simulink library "lib_electric_machine2"  (Simulink 10.1)
settings: Solver=VariableStepAuto  StartTime=0.0  StopTime=10.0  RelTol=1e-3
undefined symbols (not defined in the file or in its folder): amb_tmp, fd_ratio, gb_ratio, gc_inertia, gc_map_spd, gc_map_trq, gc_max_crrnt, gc_max_trq, gc_outpwr_map, gc_overtrq_factor, gc_spd_scale, gc_trq_scale, mc_cp, mc_inertia, mc_init_tmp, mc_inpwr_map, mc_map_spd, mc_map_trq, mc_mass, mc_max_crrnt, mc_max_gen_trq, mc_max_trq, mc_overtrq_factor, mc_sarea, mc_spd_scale, mc_th_calc, mc_trq_scale, mc_tstat, veh_mass, wh_radius
undefined symbols (not defined in the file): logFlag
libraries: lib_electric_machine x1
(part 3 of 3)

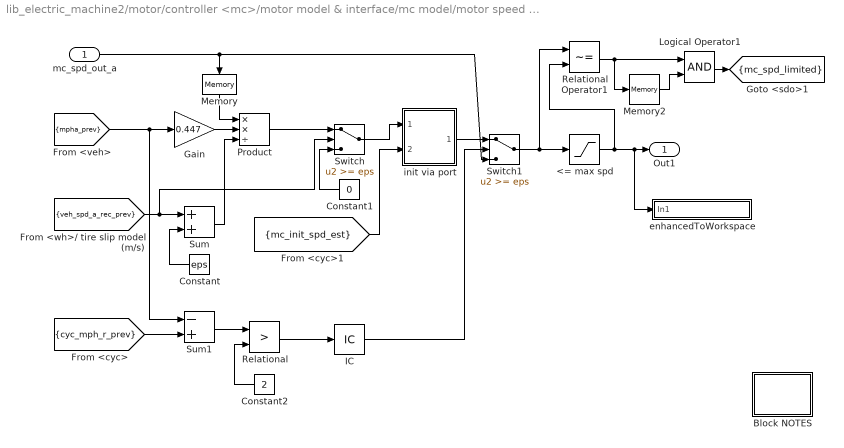
== system lib_electric_machine2/motor/controller <mc>/motor model & interface/mc model/motor speed estimator ==
  mc_spd_out_a : Inport
  <= max spd : Saturate  UpperLimit=max(mc_map_spd)*mc_spd_scale  LowerLimit=-inf
  Block NOTES : Subsystem
      mask Display: disp('Block\nNOTES')
  Constant : Constant  Value=eps
  Constant1 : Constant  Value=0
  Constant2 : Constant  Value=2
  Gain : Gain  Gain=0.447  SaturateOnIntegerOverflow=on
  IC : InitialCondition
  Logical Operator1 : Logic
  Memory : Memory
  Memory2 : Memory
  Product : Product  Inputs=**/  SaturateOnIntegerOverflow=on
  Relational : RelationalOperator  Operator=>  RndMeth=Nearest  InputSameDT=on
  Relational Operator1 : RelationalOperator  Operator=~=  RndMeth=Nearest  InputSameDT=on
  Sum : Sum  SaturateOnIntegerOverflow=on
  Sum1 : Sum  Inputs=-+  SaturateOnIntegerOverflow=on
  Switch : Switch  Threshold=eps  SaturateOnIntegerOverflow=on  InputSameDT=on
  Switch1 : Switch  Threshold=eps  SaturateOnIntegerOverflow=on  InputSameDT=on
  enhancedToWorkspace : Subsystem  mask(enhancedToWorkspace){generalName=generalName, specificName=spd_est, logFlag=logFlag}
      mask prompts: generalName "General Name [char-evaluated]"; specificName "Specific Name [char-literal]"; logFlag "Enable flag (1=on,0=off)"
      mask help: A wrapper for the Simulink "To Workspace" block that allows you to evaluate the name of the variable to log to workspace. This is useful to avoid the double logging errors that occur when you pull in two library models that attempt to log to the same variable.
      mask init:
      | enhancedToWsMaker
      settings: CopyFcn=breakLinkCopyFcn  ParentCloseFcn=breakLinkParCloseFcn
      mask Help:
      | <h2>Enhanced To Workspace Block</h2>
      | <h3>Parameters</h3>
      | <UL>
      | <li><b>General Name:</b> This is the more general name of the variable. Variables are saved to the workspace as <i>generalName_specificName</i>. Note that this is an evaluated variable. If you would like to type in the value directly, it must be surrounded with single quotes. Otherwise you can input the name of a variable containing a char string.</li>
      | <li><b>Specific Name:</b> This is the specific name of the variable. Note that this is input as a char literal (i.e., you don't need quotes).</li>
      | <li><b>Enable Flag:</b> This flag should have the value of 0 or 1. If 0, the variable will not be logged to the workspace. If 1, the variable will be logged. This is done so that variable logging can be turned off to improve speed.</li>
      | </ul>
      | <h3>Overview</h3>
      | <p>The enhanced to workspace block was put together to allow one to dynamically resolve variable names at run time in simulink. This is most powerful when used in conjunction with a masked subsystem to allow multiple instances of that masked subsytem to be used in the same model. The strategy is to set the generalName in the block mask which will allow the block to change the general name for all variable logging on the fly.
      | <h3>Helper Files</h3>
      | <p>Three m-files are required by the enhancedToWorkspace block. These files are located in the &lt; ADVISOR root &gt;/GUI directory :
      | <ul>
      | <li><i>enhancedToWsMaker.m</i> This file runs the mask initialization for the block</li>
      | <li><i>breakLinkCopyFcn.m</i> This file is used by the block callback when the simulink block is copied. It is necessary to break the link to the enhancedToWorkspace similar to the To Workspace block in order for it to be able to configure itself. (Try copying simulink's To Workspace block--it is impossible to make a link)</li>
      | <li><i>breakLinkParCloseFcn.m</i> This file is similar to the breakLinkCopyFcn and is used when a parent system is closed</li>
      | </ul>
      | <hr>
      | 
      | <p>Created 2003-Jan-21, Michael Patrick O'Keefe, NREL</p>
      mask Display: disp([generalName,'_',specificName])
  init via port : Subsystem
  Out1 : Outport
  tag scope: mc_spd_limited=scoped
  wires:
  Memory/1 -> Product/1
  [mc_init_spd_est] -> init via port/2(signal init)
  <= max spd/1 -> Relational Operator1/2, Out1/1, enhancedToWorkspace/1(In1)
  Switch1/1 -> Relational Operator1/1, <= max spd/1
  Relational Operator1/1 -> Memory2/1, Logical Operator1/1
  Logical Operator1/1 -> [mc_spd_limited]
  Memory2/1 -> Logical Operator1/2
  mc_spd_out_a/1 -> Memory/1, Switch1/3
  Product/1 -> Switch/1
  Sum/1 -> Product/3
  Gain/1 -> Product/2
  [veh_spd_a_rec_prev] -> Sum/1, Switch/2
  Constant1/1 -> Switch/3
  init via port/1(signal out) -> Switch1/1
  Constant/1 -> Sum/2
  [cyc_mph_r_prev] -> Sum1/2
  [mpha_prev] -> Gain/1, Sum1/1
  Constant2/1 -> Relational/2
  Sum1/1 -> Relational/1
  Relational/1 -> IC/1
  IC/1 -> Switch1/2
  Switch/1 -> init via port/1(signal in)

== system lib_electric_machine2/motor/controller <mc>/motor model & interface/mc model/rotor drive torque available (Nm) ==
  torque per unit input power (N-m/W) : Inport
  available input power (W) : Inport  Port=2
  Block NOTES : Subsystem
      mask Display: disp('Block\nNOTES')
  Constant2 : Constant  Value=inf
  Constant3 : Constant  Value=0
  Product : Product  SaturateOnIntegerOverflow=on
  Relational Operator : RelationalOperator  Operator=~=  RndMeth=Nearest  InputSameDT=on
  Switch : Switch  Threshold=eps  SaturateOnIntegerOverflow=on  InputSameDT=on
  rotor drive torque available : Outport  InitialOutput=0
  wires:
  Constant3/1 -> Switch/3
  Constant2/1 -> Relational Operator/2
  available input power (W)/1 -> Product/2
  Product/1 -> Switch/1
  Relational Operator/1 -> Switch/2
  Switch/1 -> rotor drive torque available/1
  torque per unit input power (N-m/W)/1 -> Product/1, Relational Operator/1

== system lib_electric_machine2/generator/ controller <gc>/GC Model/model/enforce torque limit/Block NOTES ==
  note: This block enforces the maximum torque
      | absorption capability limit of the generator.

== system lib_electric_machine2/generator/ controller <gc>/GC Model/model/limit request: controller current limit/Block NOTES ==
  note: This block prevents the generator/controller set from
      | outputting more than its maximum rated current.

== system lib_electric_machine2/motor/controller <mc>/motor model & interface/mc model/N-m drive torque per W input/Block NOTES ==
  note: This block determines the ratio of req'd rotor torque to req'd electrical input power,
      |  which is proportional to efficiency if the motor is providing torque.  This ratio is used
      | to compute actual rotor torque given some input power which may be different from
      | the req'd value.
      |
      | If the denominator, the req'd input power, is zero, this block outputs inf,
      | which is a flag used by the block .../rotor drive torque available (Nm).

== system lib_electric_machine2/motor/controller <mc>/motor model & interface/mc model/effect of inertia (Nm)/Block NOTES ==
  note: Torque required to accelerate the motor's inertia is calculated from the rate of change
      | of mc_spd_out_a.  It is no greater than the product of the maximum motor torque and
      | the fractional contribution of the motor's inertia to the total vehicle inertia.

== system lib_electric_machine2/motor/controller <mc>/motor model & interface/mc model/effect of inertia (Nm)/motor inertia as a function of total vehicle inertia (generous approximation) ==
  gear ratio : Inport
  Product : Product  Inputs=*/  SaturateOnIntegerOverflow=on
  Sum : Sum  Inputs=++|  SaturateOnIntegerOverflow=on
  engine inertia as a fraction of total vehicle inertia  (generous approximation)--denomenator : Fcn  Expr=mc_inertia*u^2
  engine inertia as a fraction of total vehicle inertia  (generous approximation)--numerator : Fcn  Expr=mc_inertia*u^2
  Out1 : Outport
  wires:
  engine inertia as a fraction of total vehicle inertia  (generous approximation)--numerator/1 -> Product/1
  Product/1 -> Out1/1
  gear ratio/1 -> engine inertia as a fraction of total vehicle inertia  (generous approximation)--numerator/1, engine inertia as a fraction of total vehicle inertia  (generous approximation)--denomenator/1
  [current_veh_mass] -> Sum/1
  engine inertia as a fraction of total vehicle inertia  (generous approximation)--denomenator/1 -> Sum/2
  Sum/1 -> Product/2

== system lib_electric_machine2/motor/controller <mc>/motor model & interface/mc model/enforce torque limit/Block NOTES ==
  note: This block enforces the maximum torque production and absorption
      | capability limits of the motor.  It assumes that exactly as much torque
      | can be absorbed as can be produced at a given speed.

== system lib_electric_machine2/motor/controller <mc>/motor model & interface/mc model/enforce torque limit/enhancedToWorkspace ==
  In1 : Inport
  To Workspace : ToWorkspace  VariableName=mc_max_trq_vec  SampleTime=-1
  wires:
  In1/1 -> To Workspace/1

== system lib_electric_machine2/motor/controller <mc>/motor model & interface/mc model/mc tmp/Block NOTES ==
  note: This block models the thermal behavior of a motor
      | and controller  with active fluid cooling.
      | The module is modeled as a single lumped thermal mass.
      | The fan is on whenever the battery temp is > the set temp.

== system lib_electric_machine2/motor/controller <mc>/motor model & interface/mc model/mc tmp/mc coolant ==
  Tcl : Inport
  "Qmc " : Inport  Port=2
  Enable : EnablePort  StatesWhenEnabling=reset
  Constant : Constant  Value=mc_tstat
  Product1 : Product  SaturateOnIntegerOverflow=on
  Relational Operator : RelationalOperator  Operator=<=  RndMeth=Nearest  InputSameDT=on
  Qmc_clt : Outport  OutputWhenDisabled=reset  InitialOutput=0
  wires:
  Relational Operator/1 -> Product1/1
  Product1/1 -> Qmc_clt/1
  "Qmc "/1 -> Product1/2
  Constant/1 -> Relational Operator/1
  Tcl/1 -> Relational Operator/2

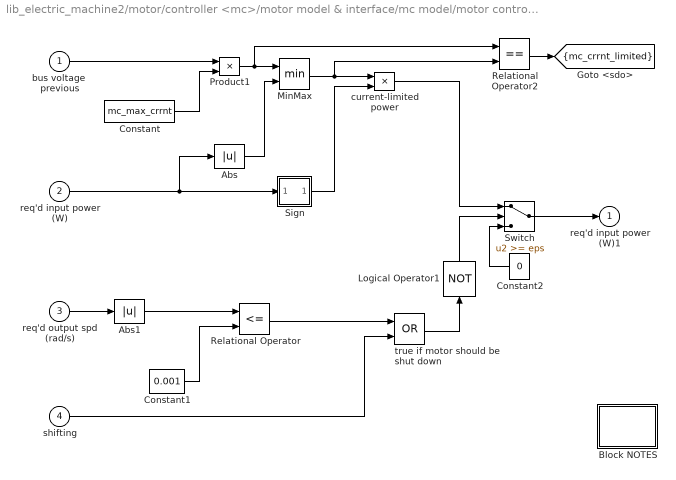
== system lib_electric_machine2/motor/controller <mc>/motor model & interface/mc model/motor controller logic interface/motor controller logic ==
  bus voltage  previous : Inport
  req'd input power (W) : Inport  Port=2
  req'd output spd (rad/s) : Inport  Port=3
  shifting : Inport  Port=4
  Abs : Abs  SaturateOnIntegerOverflow=on
  Abs1 : Abs  SaturateOnIntegerOverflow=on
  Block NOTES : Subsystem
      mask Display: disp('Block\nNOTES')
  Constant : Constant  Value=mc_max_crrnt
  Constant1 : Constant  Value=0.001
  Constant2 : Constant  Value=0
  Logical Operator1 : Logic  Operator=NOT  Inputs=1
  MinMax : MinMax  Inputs=2
  Product1 : Product  SaturateOnIntegerOverflow=on
  Relational Operator : RelationalOperator  Operator=<=  RndMeth=Nearest  InputSameDT=on
  Relational Operator2 : RelationalOperator  Operator===  RndMeth=Nearest  InputSameDT=on
  Sign : Subsystem  mask(Sign){}
      mask help: y = sign(x)
      mask Help: Sign Function:\n\t\t\ty = 1 if x > 0\n\t\t\ty = 0 if x = 0\n\t\t\ty = -1 if x < 0
      mask Display: plot(-50,-50,50,50,[-50,50],[0,0],[0,0],[-50,50],[-40,0],[-30,-30],[0,40],[30,30])
  Switch : Switch  Threshold=eps  SaturateOnIntegerOverflow=on  InputSameDT=on
  current-limited power : Product  SaturateOnIntegerOverflow=on
  true if motor should be shut down : Logic  Operator=OR
  req'd input power (W)1 : Outport  InitialOutput=0
  tag scope: mc_crrnt_limited=scoped
  wires:
  Abs1/1 -> Relational Operator/1
  req'd output spd (rad/s)/1 -> Abs1/1
  Constant1/1 -> Relational Operator/2
  Relational Operator/1 -> true if motor should be shut down/1
  Relational Operator2/1 -> [mc_crrnt_limited]
  MinMax/1 -> Relational Operator2/2, current-limited power/1
  Product1/1 -> Relational Operator2/1, MinMax/1
  current-limited power/1 -> Switch/1
  Switch/1 -> req'd input power (W)1/1
  Constant2/1 -> Switch/3
  Sign/1(out_1) -> current-limited power/2
  Abs/1 -> MinMax/2
  req'd input power (W)/1 -> Sign/1(in_1), Abs/1
  Constant/1 -> Product1/2
  bus voltage  previous/1 -> Product1/1
  true if motor should be shut down/1 -> Logical Operator1/1
  Logical Operator1/1 -> Switch/2
  shifting/1 -> true if motor should be shut down/2

== system lib_electric_machine2/motor/controller <mc>/motor model & interface/mc model/motor speed estimator/Block NOTES ==
  note: The requested motor speed is replaced by an estimate of the
      | motor's previous speed, for loss and max. torque calculations,
      | whenever the vehicle missed the trace by more than 1 mph
      | on the last time step.

== system lib_electric_machine2/motor/controller <mc>/motor model & interface/mc model/motor speed estimator/enhancedToWorkspace ==
  In1 : Inport
  To Workspace : ToWorkspace  VariableName=mc_spd_est  SampleTime=-1
  wires:
  In1/1 -> To Workspace/1

== system lib_electric_machine2/motor/controller <mc>/motor model & interface/mc model/motor speed estimator/init via port ==
  signal in : Inport
  signal init : Inport  Port=2
  Constant : Constant
  IC : InitialCondition  Value=0
  Switch : Switch  Threshold=0.5  SaturateOnIntegerOverflow=on  InputSameDT=on
  signal out : Outport
  wires:
  signal in/1 -> Switch/1
  Constant/1 -> IC/1
  IC/1 -> Switch/2
  Switch/1 -> signal out/1
  signal init/1 -> Switch/3

== system lib_electric_machine2/motor/controller <mc>/motor model & interface/mc model/rotor drive torque available (Nm)/Block NOTES ==
  note: This block computes the actual rotor torque given the actual motor input power and
      | the ratio (req'd rotor torque)/(req'd input power).
      |
      | If the above ratio has the value inf, which implies that the req'd input power is zero,
      | then the actual rotor torque is assumed to be zero.  This is not reflective of reality, of course:
      | with zero input power, the rotor torque would be the motor spin-loss torque at the given speed.
      | Because this simplification occurs only when req'd input power is zero, it does not.
      | affect fuel economy or max effort acceleration calculations.

== system lib_electric_machine2/motor/controller <mc>/motor model & interface/mc model/motor controller logic interface/motor controller logic/Block NOTES ==
  note: This block models a motor/controller's logic, modulating the power input requirement as follows:
      | - enforcing the maximum current limit of the motor/controller
      | - shutting the motor off if the average speed over the time step ==0
      | - shutting the motor off if the transmission is shifting.

== system lib_electric_machine2/motor/controller <mc>/motor model & interface/mc model/motor controller logic interface/motor controller logic/Sign ==
  in_1 : Inport
  Constant : Constant  Value=0
  Relational Operator : RelationalOperator  Operator=>  RndMeth=Nearest  InputSameDT=on
  Relational Operator1 : RelationalOperator  Operator=<  RndMeth=Nearest  InputSameDT=on
  Sum : Sum  Inputs=+-  SaturateOnIntegerOverflow=on
  out_1 : Outport  InitialOutput=0
  wires:
  in_1/1 -> Relational Operator/1, Relational Operator1/1
  Constant/1 -> Relational Operator1/2, Relational Operator/2
  Relational Operator1/1 -> Sum/2
  Relational Operator/1 -> Sum/1
  Sum/1 -> out_1/1
